simulink model "Pi_controller"  (R2020b)
settings: Solver=VariableStepAuto  StartTime=0.0  StopTime=10.0  RelTol=1e-3
model workspace (MAT data in the model file):
  Ki = 40
  Kp = 1500
settings Model: Creator=user  LastModifiedBy=user

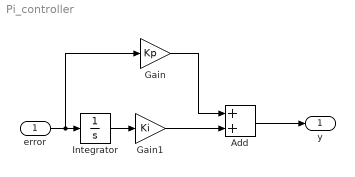
== system Pi_controller ==
  error : Inport  OutDataTypeStr=double  PortDimensions=1  SampleTime=0
  Add : Sum
  Gain : Gain  Gain=Kp
  Gain1 : Gain  Gain=Ki
  Integrator : Integrator
  y : Outport  OutDataTypeStr=double  PortDimensions=1  SampleTime=0
  wires:
  Integrator/1 -> Gain1/1
  Add/1 -> y/1
  Gain/1 -> Add/1
  Gain1/1 -> Add/2
  error/1 -> Integrator/1, Gain/1
